simulink model "winter_simulink"  (R2022b)
settings: Solver=FixedStepAuto  StartTime=0.0  StopTime=300  FixedStep=sample_time/10  RelTol=1e-3
values from neighbouring files (symbols this model uses):
  cP_vs_lambda = load('Cp_Lambda.txt')    [main.m]
  rho = 1.225    [main.m]
  sample_time = wind_speed(2,1) - wind_speed(1, 1)    [main.m]
undefined symbols (not defined in the file or in its folder): generator, omega_r, rotor
settings Model: Creator=Niccolò  LastModifiedBy=user
settings ModelReferenceCC: EnableRefExpFcnMdlSchedulingChecks=on

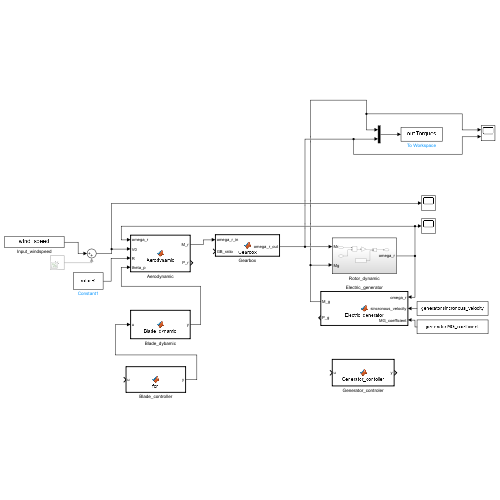
[thumbnail: Simulink's stored preview of the top-level diagram]
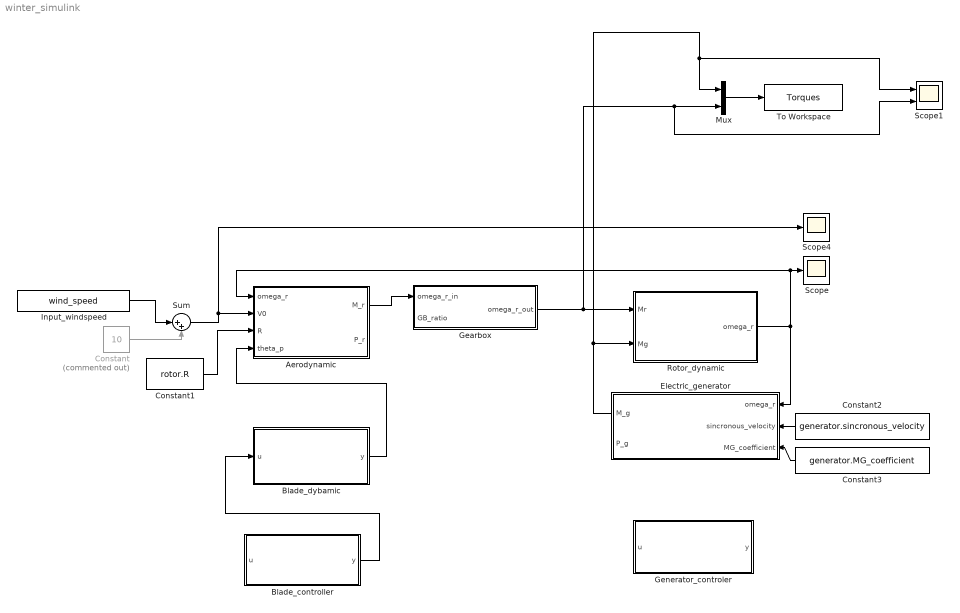
== system winter_simulink ==
  Aerodynamic : MATLAB Function  TreatAsAtomicUnit=on
  Blade_controller : MATLAB Function  TreatAsAtomicUnit=on
  Blade_dybamic : MATLAB Function  TreatAsAtomicUnit=on
  Constant : Constant  Commented=on  Value=10
  Constant1 : Constant  Value=rotor.R
  Constant2 : Constant  Value=generator.sincronous_velocity
  Constant3 : Constant  Value=generator.MG_coefficient
  Electric_generator : MATLAB Function  TreatAsAtomicUnit=on
  Gearbox : MATLAB Function  TreatAsAtomicUnit=on
  Generator_controler : MATLAB Function  TreatAsAtomicUnit=on
  Input_windspeed : FromWorkspace  VariableName=wind_speed  SampleTime=sample_time
  Mux : Mux  Inputs=2
  Rotor_dynamic : Subsystem
  Scope : Scope
  Scope1 : Scope  NumInputPorts=2
  Scope4 : Scope
  Sum : Sum  Inputs=|++
  To Workspace : ToWorkspace  VariableName=Torques  SampleTime=-1
  wires:
  Aerodynamic/1(M_r) -> Gearbox/1(omega_r_in)
  Electric_generator/1(M_g) -> Mux/1, Scope1/1, Rotor_dynamic/2(Mg)
  Input_windspeed/1 -> Sum/1
  Constant/1 -> Sum/2
  Sum/1 -> Scope4/1, Aerodynamic/2(V0)
  Rotor_dynamic/1(omega_r) -> Aerodynamic/1(omega_r), Scope/1, Electric_generator/1(omega_r)
  Mux/1 -> To Workspace/1
  Constant1/1 -> Aerodynamic/3(R)
  Constant2/1 -> Electric_generator/2(sincronous_velocity)
  Constant3/1 -> Electric_generator/3(MG_coefficient)
  Gearbox/1(omega_r_out) -> Rotor_dynamic/1(Mr), Mux/2, Scope1/2
  Blade_dybamic/1(y) -> Aerodynamic/4(theta_p)
  Blade_controller/1(y) -> Blade_dybamic/1(u)

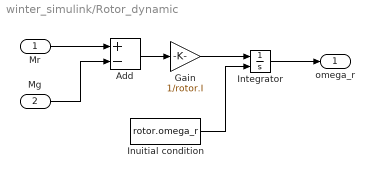
== system winter_simulink/Rotor_dynamic ==
  Mr : Inport
  Mg : Inport  Port=2
  Add : Sum  Inputs=+-
  Gain : Gain  Gain=1/rotor.I
  Integrator : Integrator  InitialConditionSource=external  InitialCondition=omega_r
  Inuitial condition : Constant  Value=rotor.omega_r
  omega_r : Outport
  wires:
  Add/1 -> Gain/1
  Gain/1 -> Integrator/1
  Mr/1 -> Add/1
  Integrator/1 -> omega_r/1
  Mg/1 -> Add/2
  Inuitial condition/1 -> Integrator/2

== matlab function winter_simulink/Gearbox ==
  data: omega_r_in input; omega_r_out output; GB_ratio input
function omega_r_out = Gearbox(omega_r_in, GB_ratio)

omega_r_out = omega_r_in*GB_ratio;

== matlab function winter_simulink/Aerodynamic ==
  data: omega_r input; V0 input; M_r output; P_r output; rho parameter; cP_vs_lambda parameter; R input; theta_p input
function [M_r, P_r] = Aerodynamic(omega_r, V0, rho, cP_vs_lambda, R, ...
    theta_p) 

lambda = omega_r*R/V0; % tip speed ratio
cP = interp1(cP_vs_lambda(:,1), cP_vs_lambda(:,2), lambda); % interpolate the table

P_r = 0.5*rho*V0^3*pi*R^2*cP; % rotor power [W]
M_r = P_r/omega_r; % rotor torque [Nm]

== matlab function winter_simulink/Electric_generator ==
  data: omega_r input; M_g output; P_g output; sincronous_velocity input; MG_coefficient input
function [M_g, P_g] = Electric_generator(omega_r, sincronous_velocity, ... 
MG_coefficient)

if omega_r < sincronous_velocity
  M_g = 0;
else
  M_g = MG_coefficient*(omega_r - sincronous_velocity);
end

P_g = M_g*omega_r;

== matlab function winter_simulink/Blade_dybamic ==
  data: u input; y output
function y = Blade_dynamic(u)

y = u;

== matlab function winter_simulink/Blade_controller ==
  data: u input; y output
function y = fcn(u)

y = u;

== matlab function winter_simulink/Generator_controler ==
  data: u input; y output
function y = Generator_contoller(u)

y = u;
